simulink model "stilllFrame_th"  (R2018b)
settings: Solver=ode8  StartTime=0.0  StopTime=0  FixedStep=0.01  RelTol=1e-3
undefined symbols (not defined in the file or in its folder): getVal, Rec, SDTV
libraries: dotFinder_ul x4, visionconversions x3, visionsources x3, find6DOF_cl x1
settings Model: Creator=mae-ncsucore  LastModifiedBy=mae-ncsucore

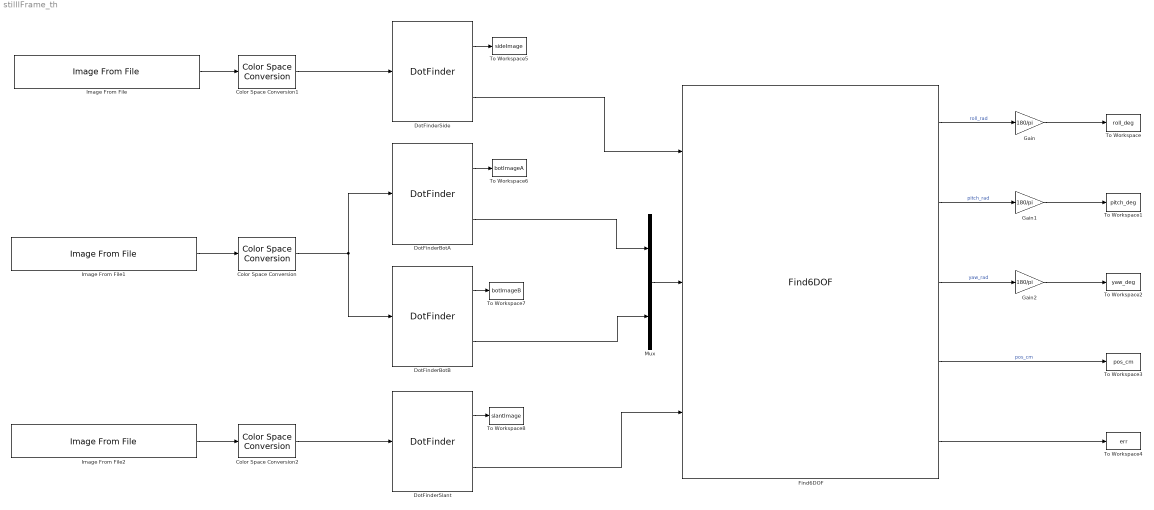
== system stilllFrame_th ==
  Color Space Conversion : visionconversions/Color Space  Conversion  conversion=Obsolete  conversionActive=R'G'B' to intensity  wp_str=D65  rec=Rec. 601 (SDTV)  sys=1125/60/2:1  imagePorts=One multidimensional signal
      settings: SourceProductName=Computer Vision System Toolbox
  Color Space Conversion1 : visionconversions/Color Space  Conversion  conversion=Obsolete  conversionActive=R'G'B' to intensity  wp_str=D65  rec=Rec. 601 (SDTV)  sys=1125/60/2:1  imagePorts=One multidimensional signal
      settings: SourceProductName=Computer Vision System Toolbox
  Color Space Conversion2 : visionconversions/Color Space  Conversion  conversion=Obsolete  conversionActive=R'G'B' to intensity  wp_str=D65  rec=Rec. 601 (SDTV)  sys=1125/60/2:1  imagePorts=One multidimensional signal
      settings: SourceProductName=Computer Vision System Toolbox
  DotFinderBotA : dotFinder_ul/DotFinder  ROIPositionHoldEnable=on  ROIPositionHoldCoordinates=[470 525]  ROIDimVec_px=[90 135]  ROIHalfDimVec_px=[45 67]  ROISplitDims_px=[1 45 ; 1 135 ; 46 44 ; 1 135]  DotOrientation=Vertical  OverlayOutput=on  ImageDimensions=[796 1487]  CrosshairPixelWidth_px=getVal('slntCrsHrWdth_px')
  DotFinderBotB : dotFinder_ul/DotFinder  ROIPositionHoldEnable=on  ROIPositionHoldCoordinates=[375 550]  ROIDimVec_px=[40 100]  ROIHalfDimVec_px=[20 50]  ROISplitDims_px=[1 40 ; 1 50 ; 1 40 ; 51 49]  DotOrientation=Horizontal  OverlayOutput=on  ImageDimensions=[796 1487]  CrosshairPixelWidth_px=getVal('slntCrsHrWdth_px')
  DotFinderSide : dotFinder_ul/DotFinder  ROIPositionHoldEnable=on  ROIPositionHoldCoordinates=[225 870]  ROIDimVec_px=[90 100]  ROIHalfDimVec_px=[45 50]  ROISplitDims_px=[1 90 ; 1 50 ; 1 90 ; 51 49]  DotOrientation=Horizontal  OverlayOutput=on  ImageDimensions=[796 1512]  CrosshairPixelWidth_px=getVal('slntCrsHrWdth_px')
  DotFinderSlant : dotFinder_ul/DotFinder  ROIPositionHoldEnable=on  ROIPositionHoldCoordinates=[500 620]  ROIDimVec_px=[50 100]  ROIHalfDimVec_px=[25 50]  ROISplitDims_px=[1 50 ; 1 50 ; 1 50 ; 51 49]  DotOrientation=Horizontal  OverlayOutput=on  ImageDimensions=[797 1506]  CrosshairPixelWidth_px=getVal('slntCrsHrWdth_px')
  Find6DOF : find6DOF_cl/Find6DOF  imageDims_px=getVal('sideImageSize_px')  initialCoMPositionVec_cm=getVal('initCoMPosVec_cm')  cameraFOVAngles_deg=getVal('cameraFOV_deg')  sideEulerAngles=[0 90 90]  sideCamPositionVec_cm=[17 45.25 33]  botEulerAngles=[0 180 180]  botCamPositionVec_cm=[15 0 -4.45]  slantEulerAngles=[0 135 180]  slantCamPositionVec_cm=[-21.6 0 -4.45]  sideSeparation_cm=2.5  sidePositionVecBF_cm=[0.091 4.54 0.878]  bottomASeparation_cm=2.2  botAPositionVecBF_cm=[2.48 0 -4.53]  bottomBSeparation_cm=2.25  botBPositionVecBG_cm=[-1 0 -4.64]
  Gain : Gain  Gain=180/pi
  Gain1 : Gain  Gain=180/pi
  Gain2 : Gain  Gain=180/pi
  Image From File : visionsources/Image From File  Tag=vipblks_nd  FileName=C:\Users\MAE-NCSUCORE\Desktop\WaterChannelControl\output\screenshots\targetScreen_Machine3_Side_Cropped.png  imagePorts=One multidimensional signal  Ts=inf  ImageDataType=Inherit from input image  Signed=on  WordLength=16  sdImageDataType=uint(8)  FractionLengthMode=User-defined  FractionLength=15  OutPortLabels=R|G|B
      settings: SourceProductName=Computer Vision System Toolbox
  Image From File1 : visionsources/Image From File  Tag=vipblks_nd  FileName=C:\Users\MAE-NCSUCORE\Desktop\WaterChannelControl\output\screenshots\targetScreen_Machine4_Bottom_Cropped.png  imagePorts=One multidimensional signal  Ts=inf  ImageDataType=Inherit from input image  Signed=on  WordLength=16  sdImageDataType=uint(8)  FractionLengthMode=User-defined  FractionLength=15  OutPortLabels=R|G|B
      settings: SourceProductName=Computer Vision System Toolbox
  Image From File2 : visionsources/Image From File  Tag=vipblks_nd  FileName=C:\Users\MAE-NCSUCORE\Desktop\WaterChannelControl\output\screenshots\targetScreen_Machine5_Slant_Cropped.png  imagePorts=One multidimensional signal  Ts=inf  ImageDataType=Inherit from input image  Signed=on  WordLength=16  sdImageDataType=uint(8)  FractionLengthMode=User-defined  FractionLength=15  OutPortLabels=R|G|B
      settings: SourceProductName=Computer Vision System Toolbox
  Mux : Mux  Inputs=2
  To Workspace : ToWorkspace  VariableName=roll_deg  SaveFormat=Timeseries  SampleTime=-1
  To Workspace1 : ToWorkspace  VariableName=pitch_deg  SaveFormat=Timeseries  SampleTime=-1
  To Workspace2 : ToWorkspace  VariableName=yaw_deg  SaveFormat=Timeseries  SampleTime=-1
  To Workspace3 : ToWorkspace  VariableName=pos_cm  SaveFormat=Timeseries  SampleTime=-1
  To Workspace4 : ToWorkspace  VariableName=err  SaveFormat=Timeseries  SampleTime=-1
  To Workspace5 : ToWorkspace  VariableName=sideImage  SampleTime=-1
  To Workspace6 : ToWorkspace  VariableName=botImageA  SampleTime=-1
  To Workspace7 : ToWorkspace  VariableName=botImageB  SampleTime=-1
  To Workspace8 : ToWorkspace  VariableName=slantImage  SampleTime=-1
  wires:
  DotFinderBotA/2 -> Mux/1
  DotFinderBotB/2 -> Mux/2
  DotFinderBotB/1 -> To Workspace7/1
  DotFinderBotA/1 -> To Workspace6/1
  DotFinderSide/1 -> To Workspace5/1
  DotFinderSlant/1 -> To Workspace8/1
  Mux/1 -> Find6DOF/2
  DotFinderSide/2 -> Find6DOF/1
  DotFinderSlant/2 -> Find6DOF/3
  Image From File1/1 -> Color Space Conversion/1
  Color Space Conversion/1 -> DotFinderBotA/1, DotFinderBotB/1
  Image From File/1 -> Color Space Conversion1/1
  Color Space Conversion1/1 -> DotFinderSide/1
  Image From File2/1 -> Color Space Conversion2/1
  Color Space Conversion2/1 -> DotFinderSlant/1
  Find6DOF/1 -> Gain/1  "roll_rad"
  Find6DOF/5 -> To Workspace4/1
  Find6DOF/4 -> To Workspace3/1  "pos_cm"
  Find6DOF/3 -> Gain2/1  "yaw_rad"
  Find6DOF/2 -> Gain1/1  "pitch_rad"
  Gain/1 -> To Workspace/1
  Gain1/1 -> To Workspace1/1
  Gain2/1 -> To Workspace2/1
